simulink model "prelab_PID"  (R2018a)
settings: Solver=VariableStepAuto  StartTime=0.0  StopTime=10  RelTol=1e-3
undefined symbols (not defined in the file or in its folder): Kd, Ki, Kp
libraries: simulink_extras x1, simulink x1
settings Model: Creator=ctf365  LastModifiedBy=ctf365

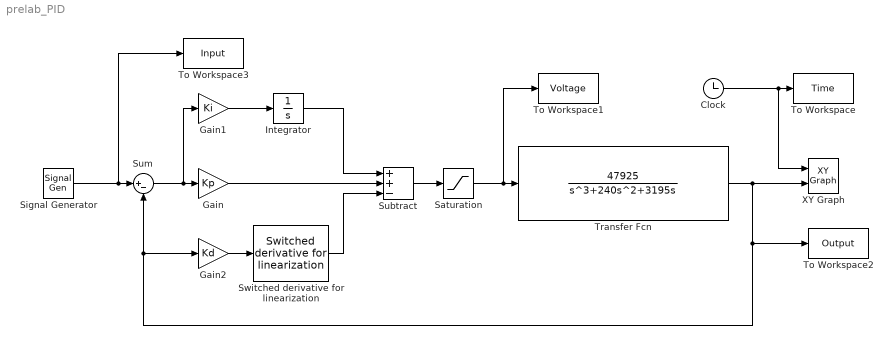
== system prelab_PID ==
  Clock : Clock
  Gain : Gain  Gain=Kp
  Gain1 : Gain  Gain=Ki
  Gain2 : Gain  Gain=Kd
  Integrator : Integrator
  Saturation : Saturate  UpperLimit=10  LowerLimit=-10
  Signal Generator : SignalGenerator  WaveForm=square  Amplitude=0.6  Frequency=0.6  Units=rad/sec
  Subtract : Sum  Inputs=++-
  Sum : Sum  Inputs=|+-
  Switched derivative for linearization : simulink_extras/Linearization/Switched derivative for linearization  switchVal=0  derivConst=100
      settings: SourceProductName=Simulink  SourceProductBaseCode=SL
  To Workspace : ToWorkspace  VariableName=Time  SaveFormat=Timeseries  SampleTime=-1
  To Workspace1 : ToWorkspace  VariableName=Voltage  SaveFormat=Timeseries  SampleTime=-1
  To Workspace2 : ToWorkspace  VariableName=Output  SaveFormat=Timeseries  SampleTime=-1
  To Workspace3 : ToWorkspace  VariableName=Input  SaveFormat=Timeseries  SampleTime=-1
  Transfer Fcn : TransferFcn  Numerator=[47925]  Denominator=[1 240 3195 0]
  XY Graph : simulink/Sinks/XY Graph  xmin=0  xmax=20  ymin=-1  ymax=2  st=-1
  wires:
  Signal Generator/1 -> To Workspace3/1, Sum/1
  Sum/1 -> Gain1/1, Gain/1
  Gain/1 -> Subtract/2
  Integrator/1 -> Subtract/1
  Switched derivative for linearization/1 -> Subtract/3
  Gain1/1 -> Integrator/1
  Gain2/1 -> Switched derivative for linearization/1
  Subtract/1 -> Saturation/1
  Saturation/1 -> To Workspace1/1, Transfer Fcn/1
  Transfer Fcn/1 -> Gain2/1, Sum/2, To Workspace2/1, XY Graph/2
  Clock/1 -> XY Graph/1, To Workspace/1
